simulink model "bassengmodell_rev2"  (R2015b)
settings: Solver=VariableStepAuto  StartTime=0.0  StopTime=t_sim  RelTol=1e-6
values from neighbouring files (symbols this model uses):
  A = V/300    (= 378541.178)    [main_1.m]    (also in main_rev2.m = 10)
  C_pv = 4.1796    [main_1.m]    (also in main_rev2.m)
  h = 5.7 + 3.8*vind    (= 24.7)    [main_1.m]    (also in main_rev2.m = 2)
  K_i = 0.0002    [main_rev2.m]
  K_p = 1000    [main_rev2.m]
  Kelvin_reg = 273.15    [main_rev2.m]
  T_0 = 15+273.15    (= 288.15)    [main_1.m]    (also in main_rev2.m = 15)
  T_om = 15+273.15    (= 288.15)    [main_1.m]    (also in main_rev2.m = 15)
  T_onsket = 30+273.15    (= 303.15)    [main_1.m]    (also in main_rev2.m = 30)
  time_delay = 60    [main_rev2.m]
  V = 30000*3785.41178    (= 113562353.4)    [main_1.m]    (also in main_rev2.m = 20000000)
libraries: simulink x1
settings Model: Creator=Åsmund  LastModifiedBy=Åsmund

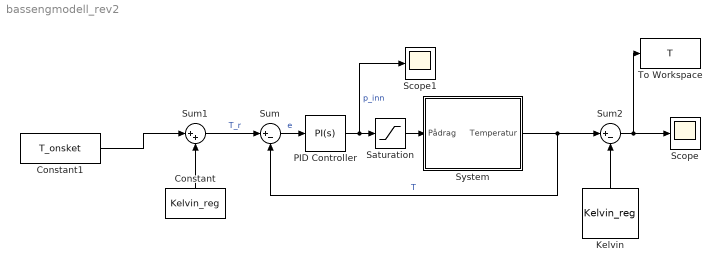
== system bassengmodell_rev2 ==
  Constant : Constant  Value=Kelvin_reg
  Constant1 : Constant  Value=T_onsket
  Kelvin : Constant  Value=Kelvin_reg
  PID Controller : simulink/Continuous/PID Controller  Controller=PI  TimeDomain=Continuous-time  SampleTime=-1  IntegratorMethod=Forward Euler  FilterMethod=Forward Euler  Form=Parallel  UseFilter=on  ControllerParametersSource=internal  P=K_p  I=K_i  D=0  N=100  InitialConditionSource=internal  InitialConditionForIntegrator=0  InitialConditionForFilter=0  ExternalReset=none  LimitOutput=off  UpperSaturationLimit=inf  LowerSaturationLimit=-inf  LinearizeAsGain=on  AntiWindupMode=none  Kb=1  TrackingMode=off  Kt=1  PParamMin=[]  PParamMax=[]  IParamMin=[]  IParamMax=[]  DParamMin=[]  DParamMax=[]  NParamMin=[]  NParamMax=[]  KbParamMin=[]  KbParamMax=[]  KtParamMin=[]  KtParamMax=[]  POutMin=[]  POutMax=[]  IOutMin=[]  IOutMax=[]  DOutMin=[]  DOutMax=[]  NOutMin=[]  NOutMax=[]  KbOutMin=[]  KbOutMax=[]  KtOutMin=[]  KtOutMax=[]  IntegratorOutMin=[]  IntegratorOutMax=[]  FilterOutMin=[]  FilterOutMax=[]  SumOutMin=[]  SumOutMax=[]  SumI1OutMin=[]  SumI1OutMax=[]  SumI2OutMin=[]  SumI2OutMax=[]  SumI3OutMin=[]  SumI3OutMax=[]  SumDOutMin=[]  SumDOutMax=[]  SaturationOutMin=[]  SaturationOutMax=[]  IntegratorContinuousStateAttributes=''  IntegratorStateMustResolveToSignalObject=off  IntegratorRTWStateStorageClass=Auto  FilterContinuousStateAttributes=''  FilterStateMustResolveToSignalObject=off  FilterRTWStateStorageClass=Auto  DifferentiatorICPrevScaledInput=0  DifferentiatorOutMin=[]  DifferentiatorOutMax=[]
  Saturation : Saturate  UpperLimit=inf  LowerLimit=0
  Scope : Scope
  Scope1 : Scope
  Sum : Sum  Inputs=|+-
  Sum1 : Sum  Inputs=|++
  Sum2 : Sum  Inputs=|+-
  System : Subsystem
  To Workspace : ToWorkspace  VariableName=T  SaveFormat=Timeseries  SampleTime=-1
  wires:
  PID Controller/1 -> Saturation/1, Scope1/1  "p_inn"
  Sum/1 -> PID Controller/1  "e"
  System/1(Temperatur) -> Sum2/1, Sum/2  "T"
  Constant1/1 -> Sum1/1
  Sum1/1 -> Sum/1  "T_r"
  Constant/1 -> Sum1/2
  Sum2/1 -> To Workspace/1, Scope/1
  Kelvin/1 -> Sum2/2
  Saturation/1 -> System/1(Pådrag)

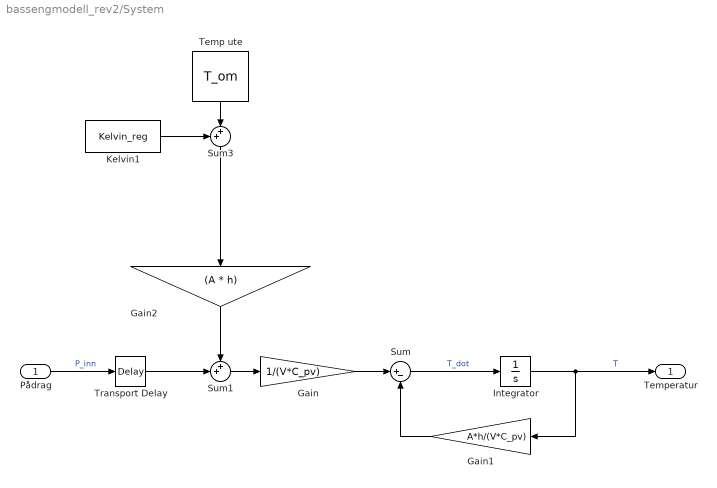
== system bassengmodell_rev2/System ==
  Pådrag : Inport
  Gain : Gain  Gain=1/(V*C_pv)
  Gain1 : Gain  Gain=A*h/(V*C_pv)
  Gain2 : Gain  Gain=(A * h)
  Integrator : Integrator  InitialCondition=T_0 + Kelvin_reg
  Kelvin1 : Constant  Value=Kelvin_reg
  Sum : Sum  Inputs=|+-
  Sum1 : Sum  Inputs=++|
  Sum3 : Sum  Inputs=++|
  Temp ute : Constant  Value=T_om
  Transport Delay : TransportDelay  DelayTime=time_delay
  Temperatur : Outport
  wires:
  Integrator/1 -> Temperatur/1, Gain1/1  "T"
  Sum/1 -> Integrator/1  "T_dot"
  Gain/1 -> Sum/1
  Gain1/1 -> Sum/2
  Sum1/1 -> Gain/1
  Gain2/1 -> Sum1/1
  Temp ute/1 -> Sum3/2
  Kelvin1/1 -> Sum3/1
  Sum3/1 -> Gain2/1
  Transport Delay/1 -> Sum1/2
  Pådrag/1 -> Transport Delay/1  "P_inn"
